simulink model "EnergyMonitoring7d"  (R2024a)
settings: Solver=VariableStepAuto  StartTime=0.0  StopTime=604800  RelTol=1e-3
settings Model: Creator=dogba  LastModifiedBy=dogba

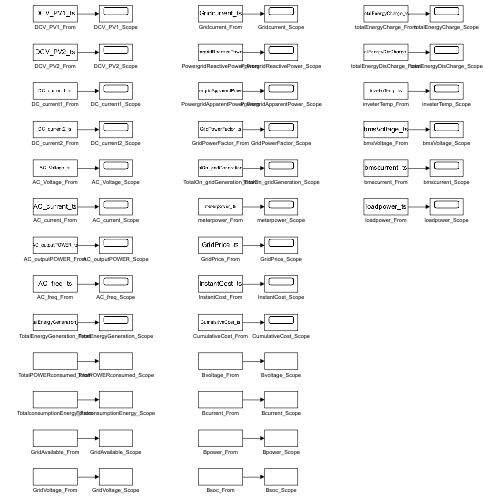
[thumbnail: Simulink's stored preview of the top-level diagram]
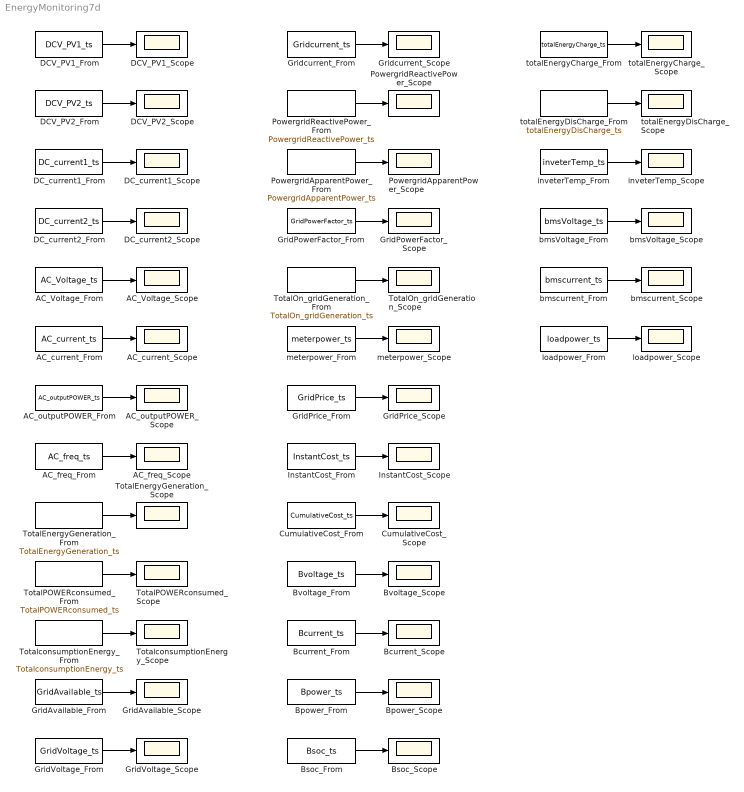
== system EnergyMonitoring7d ==
  AC_Voltage_From : FromWorkspace  VariableName=AC_Voltage_ts
  AC_Voltage_Scope : Scope
  AC_current_From : FromWorkspace  VariableName=AC_current_ts
  AC_current_Scope : Scope
  AC_freq_From : FromWorkspace  VariableName=AC_freq_ts
  AC_freq_Scope : Scope
  AC_outputPOWER_From : FromWorkspace  VariableName=AC_outputPOWER_ts
  AC_outputPOWER_Scope : Scope
  Bcurrent_From : FromWorkspace  VariableName=Bcurrent_ts
  Bcurrent_Scope : Scope
  Bpower_From : FromWorkspace  VariableName=Bpower_ts
  Bpower_Scope : Scope
  Bsoc_From : FromWorkspace  VariableName=Bsoc_ts
  Bsoc_Scope : Scope
  Bvoltage_From : FromWorkspace  VariableName=Bvoltage_ts
  Bvoltage_Scope : Scope
  CumulativeCost_From : FromWorkspace  VariableName=CumulativeCost_ts
  CumulativeCost_Scope : Scope
  DCV_PV1_From : FromWorkspace  VariableName=DCV_PV1_ts
  DCV_PV1_Scope : Scope
  DCV_PV2_From : FromWorkspace  VariableName=DCV_PV2_ts
  DCV_PV2_Scope : Scope
  DC_current1_From : FromWorkspace  VariableName=DC_current1_ts
  DC_current1_Scope : Scope
  DC_current2_From : FromWorkspace  VariableName=DC_current2_ts
  DC_current2_Scope : Scope
  GridAvailable_From : FromWorkspace  VariableName=GridAvailable_ts
  GridAvailable_Scope : Scope
  GridPowerFactor_From : FromWorkspace  VariableName=GridPowerFactor_ts
  GridPowerFactor_Scope : Scope
  GridPrice_From : FromWorkspace  VariableName=GridPrice_ts
  GridPrice_Scope : Scope
  GridVoltage_From : FromWorkspace  VariableName=GridVoltage_ts
  GridVoltage_Scope : Scope
  Gridcurrent_From : FromWorkspace  VariableName=Gridcurrent_ts
  Gridcurrent_Scope : Scope
  InstantCost_From : FromWorkspace  VariableName=InstantCost_ts
  InstantCost_Scope : Scope
  PowergridApparentPower_From : FromWorkspace  VariableName=PowergridApparentPower_ts
  PowergridApparentPower_Scope : Scope
  PowergridReactivePower_From : FromWorkspace  VariableName=PowergridReactivePower_ts
  PowergridReactivePower_Scope : Scope
  TotalEnergyGeneration_From : FromWorkspace  VariableName=TotalEnergyGeneration_ts
  TotalEnergyGeneration_Scope : Scope
  TotalOn_gridGeneration_From : FromWorkspace  VariableName=TotalOn_gridGeneration_ts
  TotalOn_gridGeneration_Scope : Scope
  TotalPOWERconsumed_From : FromWorkspace  VariableName=TotalPOWERconsumed_ts
  TotalPOWERconsumed_Scope : Scope
  TotalconsumptionEnergy_From : FromWorkspace  VariableName=TotalconsumptionEnergy_ts
  TotalconsumptionEnergy_Scope : Scope
  bmsVoltage_From : FromWorkspace  VariableName=bmsVoltage_ts
  bmsVoltage_Scope : Scope
  bmscurrent_From : FromWorkspace  VariableName=bmscurrent_ts
  bmscurrent_Scope : Scope
  inveterTemp_From : FromWorkspace  VariableName=inveterTemp_ts
  inveterTemp_Scope : Scope
  loadpower_From : FromWorkspace  VariableName=loadpower_ts
  loadpower_Scope : Scope
  meterpower_From : FromWorkspace  VariableName=meterpower_ts
  meterpower_Scope : Scope
  totalEnergyCharge_From : FromWorkspace  VariableName=totalEnergyCharge_ts
  totalEnergyCharge_Scope : Scope
  totalEnergyDisCharge_From : FromWorkspace  VariableName=totalEnergyDisCharge_ts
  totalEnergyDisCharge_Scope : Scope
  wires:
  DCV_PV1_From/1 -> DCV_PV1_Scope/1
  DCV_PV2_From/1 -> DCV_PV2_Scope/1
  DC_current1_From/1 -> DC_current1_Scope/1
  DC_current2_From/1 -> DC_current2_Scope/1
  AC_Voltage_From/1 -> AC_Voltage_Scope/1
  AC_current_From/1 -> AC_current_Scope/1
  AC_outputPOWER_From/1 -> AC_outputPOWER_Scope/1
  AC_freq_From/1 -> AC_freq_Scope/1
  TotalEnergyGeneration_From/1 -> TotalEnergyGeneration_Scope/1
  TotalPOWERconsumed_From/1 -> TotalPOWERconsumed_Scope/1
  TotalconsumptionEnergy_From/1 -> TotalconsumptionEnergy_Scope/1
  GridAvailable_From/1 -> GridAvailable_Scope/1
  GridVoltage_From/1 -> GridVoltage_Scope/1
  Gridcurrent_From/1 -> Gridcurrent_Scope/1
  PowergridReactivePower_From/1 -> PowergridReactivePower_Scope/1
  PowergridApparentPower_From/1 -> PowergridApparentPower_Scope/1
  GridPowerFactor_From/1 -> GridPowerFactor_Scope/1
  TotalOn_gridGeneration_From/1 -> TotalOn_gridGeneration_Scope/1
  meterpower_From/1 -> meterpower_Scope/1
  GridPrice_From/1 -> GridPrice_Scope/1
  InstantCost_From/1 -> InstantCost_Scope/1
  CumulativeCost_From/1 -> CumulativeCost_Scope/1
  Bvoltage_From/1 -> Bvoltage_Scope/1
  Bcurrent_From/1 -> Bcurrent_Scope/1
  Bpower_From/1 -> Bpower_Scope/1
  Bsoc_From/1 -> Bsoc_Scope/1
  totalEnergyCharge_From/1 -> totalEnergyCharge_Scope/1
  totalEnergyDisCharge_From/1 -> totalEnergyDisCharge_Scope/1
  inveterTemp_From/1 -> inveterTemp_Scope/1
  bmsVoltage_From/1 -> bmsVoltage_Scope/1
  bmscurrent_From/1 -> bmscurrent_Scope/1
  loadpower_From/1 -> loadpower_Scope/1
